simulink model "msdDoubleVectorized"  (R2020b)
settings: Solver=VariableStepAuto  StartTime=0.0  StopTime=20  RelTol=1e-6
settings Model: Creator=Rocksmithed  LastModifiedBy=Rocksmithed

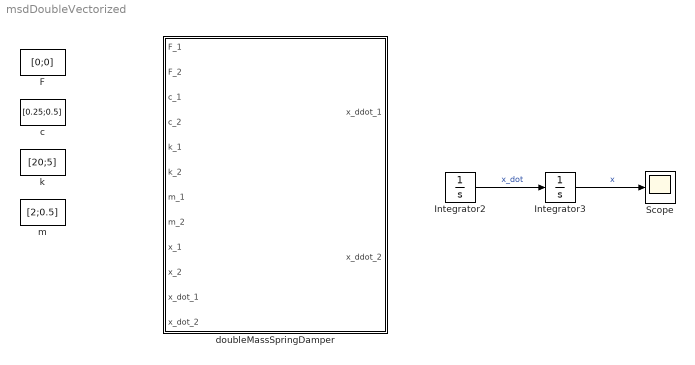
== system msdDoubleVectorized ==
  F : Constant  Value=[0;0]
  Integrator2 : Integrator  InitialCondition=[0;8]
  Integrator3 : Integrator  InitialCondition=[0;0]
  Scope : Scope
  c : Constant  Value=[0.25;0.5]
  doubleMassSpringDamper : MATLAB Function  TreatAsAtomicUnit=on
  k : Constant  Value=[20;5]
  m : Constant  Value=[2;0.5]
  wires:
  Integrator2/1 -> Integrator3/1  "x_dot"
  Integrator3/1 -> Scope/1  "x"

== matlab function msdDoubleVectorized/doubleMassSpringDamper ==
  data: F_1 input; x_ddot_1 output; F_2 input; c_1 input; c_2 input; k_1 input; k_2 input; m_1 input; m_2 input; x_1 input; x_2 input; x_dot_1 input; x_dot_2 input; x_ddot_2 output
function [x_ddot_1,x_ddot_2] = doubleMassSpringDamper(F_1,F_2,c_1,c_2,k_1,k_2,m_1,m_2,x_1,x_2,x_dot_1,x_dot_2)
%#codegen


x_ddot_1 = -(-F_1+c_1.*x_dot_1+k_1.*x_1+c_2.*(x_dot_1-x_dot_2)+k_2.*(x_1-x_2))./m_1;
x_ddot_2 = (F_2+c_2.*(x_dot_1-x_dot_2)+k_2.*(x_1-x_2))./m_2;
